simulink library "pacejka_trans"  (R2018b)
settings: Solver=ode45  StartTime=0.0  StopTime=10.0  RelTol=1e-3  EnableMultiTasking=on
undefined symbols (not defined in the file): DiscIntNeverNeededParam, par_TIR
libraries: simulink x2, $bdroot x1
(part 2 of 2)

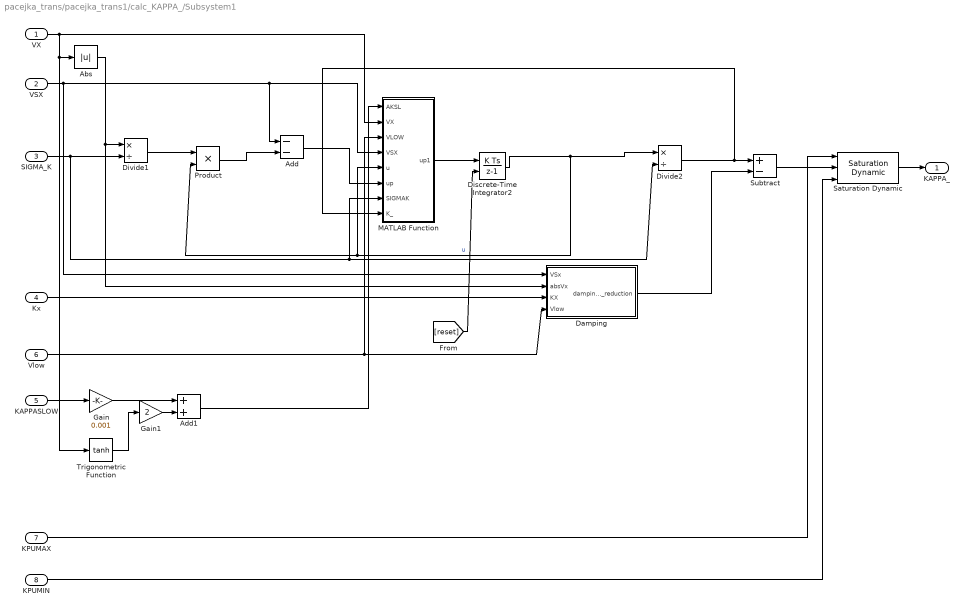
== system pacejka_trans/pacejka_trans1/calc_KAPPA_/Subsystem1 ==
  VX : Inport
  VSX : Inport  Port=2
  SIGMA_K : Inport  Port=3
  Kx : Inport  Port=4
  KAPPASLOW : Inport  Port=5
  Vlow : Inport  Port=6
  KPUMAX : Inport  Port=7
  KPUMIN : Inport  Port=8
  Abs : Abs
  Add : Sum  Inputs=--
  Add1 : Sum
  Damping : Subsystem
  Discrete-Time Integrator2 : DiscreteIntegrator  ExternalReset=sampled level  SampleTime=-1  ICPrevOutput=DiscIntNeverNeededParam  ICPrevScaledInput=DiscIntNeverNeededParam
  Divide1 : Product  Inputs=*/
  Divide2 : Product  Inputs=*/
  Gain : Gain  Gain=0.001
  Gain1 : Gain  Gain=2
  MATLAB Function : MATLAB Function  TreatAsAtomicUnit=on
  Product : Product  RndMeth=Zero
  Saturation Dynamic : simulink/Discontinuities/Saturation Dynamic  OutMin=[]  OutMax=[]  OutDataTypeStr=Inherit: Same as second input  OutDataType=fixdt(1, 16)  OutScaling=2^-10  DoSatur=off
  Subtract : Sum  Inputs=+-
  Trigonometric Function : Trigonometry  Operator=tanh
  KAPPA_ : Outport
  wires:
  Saturation Dynamic/1 -> KAPPA_/1
  KPUMIN/1 -> Saturation Dynamic/3
  KPUMAX/1 -> Saturation Dynamic/1
  MATLAB Function/1(up1) -> Discrete-Time Integrator2/1
  Add/1 -> MATLAB Function/6(up)
  Vlow/1 -> MATLAB Function/3(VLOW), Damping/4(Vlow)
  KAPPASLOW/1 -> Gain/1
  Kx/1 -> Damping/3(KX)
  Product/1 -> Add/2
  Divide1/1 -> Product/1
  Abs/1 -> Damping/2(absVx), Divide1/1
  VSX/1 -> MATLAB Function/4(VSX), Add/1, Damping/1(VSx)
  Discrete-Time Integrator2/1 -> Product/2, MATLAB Function/5(u), Divide2/1  "u"
  VX/1 -> Abs/1, Trigonometric Function/1, MATLAB Function/2(VX)
  SIGMA_K/1 -> Divide1/2, MATLAB Function/7(SIGMAK), Divide2/2
  Subtract/1 -> Saturation Dynamic/2
  Damping/1(damping_reduction) -> Subtract/2
  Divide2/1 -> Subtract/1, MATLAB Function/8(K_)
  Gain/1 -> Add1/1
  Trigonometric Function/1 -> Gain1/1
  Gain1/1 -> Add1/2
  Add1/1 -> MATLAB Function/1(AKSL)
  [reset] -> Discrete-Time Integrator2/2

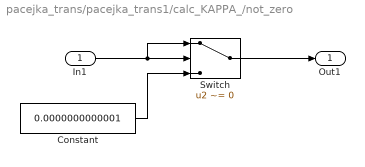
== system pacejka_trans/pacejka_trans1/calc_KAPPA_/not_zero ==
  In1 : Inport
  Constant : Constant  Value=0.0000000000001
  Switch : Switch  Criteria=u2 ~= 0
  Out1 : Outport
  wires:
  In1/1 -> Switch/1, Switch/2
  Constant/1 -> Switch/3
  Switch/1 -> Out1/1

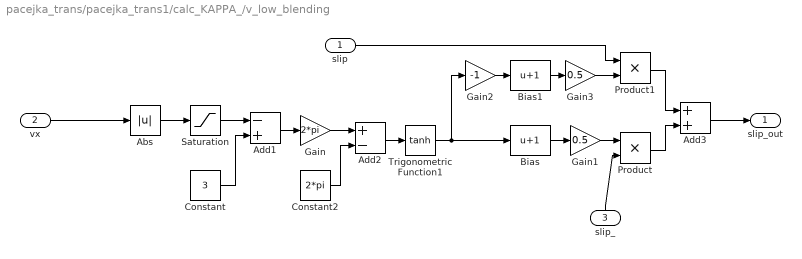
== system pacejka_trans/pacejka_trans1/calc_KAPPA_/v_low_blending  ==
  slip : Inport
  vx : Inport  Port=2
  slip_ : Inport  Port=3
  Abs : Abs
  Add1 : Sum  Inputs=-+
  Add2 : Sum  Inputs=+-
  Add3 : Sum
  Bias : Bias  Bias=1
  Bias1 : Bias  Bias=1
  Constant : Constant  Value=3
  Constant2 : Constant  Value=2*pi
  Gain : Gain  Gain=2*pi
  Gain1 : Gain  Gain=0.5
  Gain2 : Gain  Gain=-1
  Gain3 : Gain  Gain=0.5
  Product : Product
  Product1 : Product
  Saturation : Saturate  UpperLimit=3  LowerLimit=0
  Trigonometric Function1 : Trigonometry  Operator=tanh
  slip_out : Outport
  wires:
  Abs/1 -> Saturation/1
  Constant2/1 -> Add2/2
  Constant/1 -> Add1/2
  Gain/1 -> Add2/1
  Saturation/1 -> Add1/1
  Add2/1 -> Trigonometric Function1/1
  Add1/1 -> Gain/1
  Gain2/1 -> Bias1/1
  Gain1/1 -> Product/1
  Bias1/1 -> Gain3/1
  Product1/1 -> Add3/1
  Add3/1 -> slip_out/1
  Bias/1 -> Gain1/1
  Gain3/1 -> Product1/2
  Product/1 -> Add3/2
  slip/1 -> Product1/1
  Trigonometric Function1/1 -> Gain2/1, Bias/1
  slip_/1 -> Product/2
  vx/1 -> Abs/1

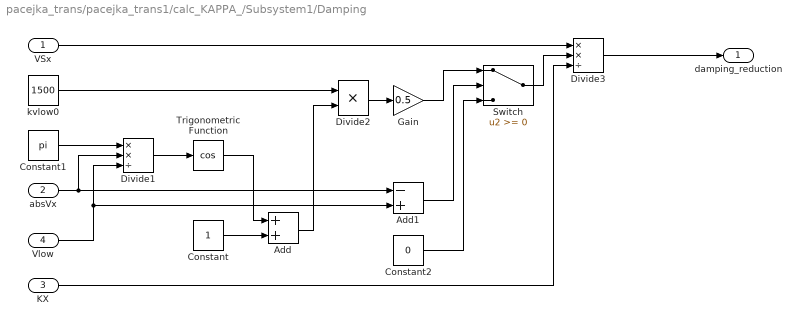
== system pacejka_trans/pacejka_trans1/calc_KAPPA_/Subsystem1/Damping ==
  VSx : Inport
  absVx : Inport  Port=2
  KX : Inport  Port=3
  Vlow : Inport  Port=4
  Add : Sum
  Add1 : Sum  Inputs=-+
  Constant : Constant
  Constant1 : Constant  Value=pi
  Constant2 : Constant  Value=0
  Divide1 : Product  Inputs=**/
  Divide2 : Product  Inputs=**
  Divide3 : Product  Inputs=**/
  Gain : Gain  Gain=0.5
  Switch : Switch
  Trigonometric Function : Trigonometry  Operator=cos
  kvlow0 : Constant  Value=1500
  damping_reduction : Outport
  wires:
  KX/1 -> Divide3/3
  Constant2/1 -> Switch/3
  Add1/1 -> Switch/2
  Divide3/1 -> damping_reduction/1
  Divide2/1 -> Gain/1
  VSx/1 -> Divide3/1
  Add/1 -> Divide2/2
  Divide1/1 -> Trigonometric Function/1
  Vlow/1 -> Add1/2, Divide1/3
  absVx/1 -> Add1/1, Divide1/2
  Constant1/1 -> Divide1/1
  Constant/1 -> Add/2
  Trigonometric Function/1 -> Add/1
  kvlow0/1 -> Divide2/1
  Gain/1 -> Switch/1
  Switch/1 -> Divide3/2

== matlab function pacejka_trans/pacejka_trans1/MATLAB Function ==
  data: RSTAT output; FZ input; OMEGA input; VX input; VSX output; VERTICAL_STIFFNESS input; FNOMIN input; UNLOADED_RADIUS input; BREFF input; DREFF input; FREFF input; RE output
function [RSTAT,VSX,RE] = longitudinal_slip_speed(FZ,OMEGA,VX,VERTICAL_STIFFNESS,FNOMIN,UNLOADED_RADIUS,BREFF,DREFF,FREFF)

RHO = FZ/VERTICAL_STIFFNESS;
RHOFZ0 = FNOMIN/VERTICAL_STIFFNESS;
RHOD = RHO/RHOFZ0;

RE = UNLOADED_RADIUS-RHOFZ0*(DREFF*atan(BREFF*RHOD)+FREFF*RHOD);
VSX = VX-OMEGA*RE;
RSTAT=UNLOADED_RADIUS-RHO;

end

== matlab function pacejka_trans/pacejka_trans1/calc_forces ==
  data: FZ input; KAPPA input; ALPHA input; GAMMA input; VX input; IP input; FNOMIN input; UNLOADED_RADIUS input; LONGVL input; LOADINDEX input; LFZO input; FX output; LCX input; LMUX input; LEX input; LKX input; LHX input; LVX input; LGAX input; LCY input; LMUY input; LEY input; LKY input; LHY input; LVY input; LGAY input; LTR input; LRES input; LGAZ input; LXAL input; LYKA input; LVYKA input; LS input; LMX input; LVMX input; LMY input; PCX1 input; PDX1 input; PDX2 input; PDX3 input; PEX1 input; PEX2 input; PEX3 input; PEX4 input; PKX1 input; PKX2 input; PKX3 input; PHX1 input; PHX2 input; PVX1 input; PVX2 input; RBX1 input; RBX2 input; RCX1 input; REX1 input; REX2 input; RHX1 input; QSX1 input; QSX2 input; QSX3 input; PCY1 input; PDY1 input; PDY2 input; PDY3 input; PEY1 input; PEY2 input; PEY3 input; PEY4 input; PKY1 input; PKY2 input; PKY3 input; PHY1 input; PHY2 input; PHY3 input; PVY1 input; PVY2 input; PVY3 input; PVY4 input; RBY1 input; RBY2 input; RBY3 input; RCY1 input; REY1 input; REY2 input; RHY1 input; RHY2 input; RVY1 input; RVY2 input; RVY3 input; RVY4 input; RVY5 input; RVY6 input; FY output; MX output; MY output; MZ output; QSY1 input; QSY2 input; QSY3 input; QSY4 input; QBZ1 input; QBZ2 input; QBZ3 input; QBZ4 input; QBZ5 input; QBZ9 input; QBZ10 input; QCZ1 input; QDZ1 input; QDZ2 input; QDZ3 input; QDZ4 input; QDZ6 input; QDZ7 input; QDZ8 input; QDZ9 input; QEZ1 input; QEZ2 input; QEZ3 input; QEZ4 input; QEZ5 input; QHZ1 input; QHZ2 input; QHZ3 input; QHZ4 input; SSZ1 input; SSZ2 input; SSZ3 input; SSZ4 input; T output; S output; Q output; c_kappa output; T_Z output; PIO input; PPX1 input; PPX2 input; PPX3 input; PPX4 input; PPY1 input; PPY2 input; PPY3 input; PPY4 input; QPZ1 input; KX output; DX output; DY output
function [FX,FY,MX,MY,MZ,T,S,Q,c_kappa,T_Z,KX,DX,DY] = magic_formula(...
    FZ, KAPPA, ALPHA, GAMMA, VX, IP,...                                         % INPUTS
    FNOMIN, UNLOADED_RADIUS, LONGVL, LOADINDEX,...                              % TIRE DATA
    LFZO,LCX,LMUX,LEX,LKX,LHX,LVX,LGAX,LCY,...                                  % SCALING FACTORS
    LMUY,LEY,LKY,LHY,LVY,LGAY,LTR,LRES,LGAZ,LXAL,LYKA,LVYKA,LS,...              % SCALING FACTORS
    LMX,LVMX,LMY,...                                                            % SCALING FACTORS
    PCX1,PDX1,PDX2,PDX3,PEX1,PEX2,PEX3,PEX4,PKX1,PKX2,PKX3,PHX1,...             % LONGITUDINAL COEFFICIENTS
    PHX2,PVX1,PVX2,RBX1,RBX2,RCX1,REX1,REX2,RHX1,...                            % LONGITUDINAL COEFFICIENTS
    QSX1,QSX2,QSX3,...                                                          % OVERTURNING COEFFICIENTS
    PCY1,PDY1,PDY2,PDY3,PEY1,PEY2,PEY3,PEY4,PKY1,...                            % LATERAL COEFFICIENTS
    PKY2,PKY3,PHY1,PHY2,PHY3,PVY1,PVY2,PVY3,PVY4,RBY1,RBY2,RBY3,RCY1,REY1,...   % LATERAL COEFFICIENTS
    REY2,RHY1,RHY2,RVY1,RVY2,RVY3,RVY4,RVY5,RVY6,...                            % LATERAL COEFFICIENTS
    QSY1,QSY2,QSY3,QSY4,...                                                     % ROLLING COEFFICIENTS
    QBZ1, QBZ2, QBZ3, QBZ4, QBZ5, QBZ9, QBZ10, QCZ1, QDZ1,...                   % ALIGNING COEFFICIENTS
    QDZ2,QDZ3,QDZ4,QDZ6,QDZ7,QDZ8,QDZ9,QEZ1,QEZ2,QEZ3,QEZ4,QEZ5,...             % ALIGNING COEFFICIENTS
    QHZ1,QHZ2,QHZ3,QHZ4,SSZ1,SSZ2,SSZ3,SSZ4,...                                 % ALIGNING COEFFICIENTS
    PIO, PPX1, PPX2, PPX3, PPX4, PPY1, PPY2, PPY3, PPY4, QPZ1)                  % PRESSURE COEFFICIENTS

%% INITIALISIERUNG

% Referenzgeschwindigkeit auf diejenige aus dem Reifenfile festlegen
VREF = LONGVL;

% calculate normalized vertical load increment dFZ
FNOMIN_ = FNOMIN.*LFZO;
dFZ = (FZ-FNOMIN_)./FNOMIN_;

% calculate normalized change in inflation pressure dPI
dPI = (IP-PIO)./PIO;

%% LONGITUDINAL

% pure slip
GAMMAX = GAMMA.*LGAX;
SHX = (PHX1+PHX2.*dFZ).*LHX;
SVX = FZ.*(PVX1+PVX2.*dFZ).*LVX.*LMUX;
KAPPAX = KAPPA+SHX;
MUX = (PDX1+PDX2.*dFZ).*(1-PDX3.*GAMMAX.^2).*LMUX.*(1+PPX3.*dPI+PPX4.*dPI.^2);
CX = PCX1.*LCX;
DX = MUX.*FZ;
EX = (PEX1+PEX2.*dFZ+PEX3.*dFZ.^2).*(1-PEX4.*sign(KAPPAX)).*LEX;
EX(EX>1) = 1;
KX = FZ.*(PKX1+PKX2.*dFZ).*exp(PKX3.*dFZ).*LKX.*(1+PPX1.*dPI+PPX2.*dPI.^2);
BX = KX./(CX.*DX);
FX0 = DX.*sin(CX.*atan(BX.*KAPPAX-EX.*(BX.*KAPPAX-atan(BX.*KAPPAX))))+SVX;

% combined slip
SHXA = RHX1;
ALPHAS = ALPHA+SHXA;
BXA = RBX1.*cos(atan(RBX2.*KAPPA)).*LXAL;
CXA = RCX1;
EXA = REX1+REX2.*dFZ;
GXA0 = cos(CXA.*atan(BXA.*SHXA-EXA.*(BXA.*SHXA-atan(BXA.*SHXA))));
GXA = cos(CXA.*atan(BXA.*ALPHAS-EXA.*(BXA.*ALPHAS-atan(BXA.*ALPHAS))))./GXA0;
FX = GXA.*FX0;

%% LATERAL

% pure slip
GAMMAY = GAMMA.*LGAY;
SHY = (PHY1+PHY2.*dFZ).*LHY+PHY3.*GAMMAY;
ALPHAY = ALPHA+SHY;
MUY = (PDY1+PDY2.*dFZ).*(1-PDY3.*GAMMAY.^2).*LMUY.*(1+PPY3.*dPI+PPY4.*dPI.^2);
SVY = FZ.*((PVY1+PVY2.*dFZ).*LVY+(PVY3+PVY4.*dFZ).*GAMMAY).*LMUY;
DY = MUY.*FZ;
CY = PCY1.*LCY;
EY = (PEY1+PEY2.*dFZ).*(1-(PEY3+PEY4.*GAMMAY).*sign(ALPHAY)).*LEY;
EY(EY>1) = 1;
KY = PKY1.*FNOMIN.*sin(2.*atan(FZ./(PKY2.*FNOMIN.*LFZO.*(1+PPY2.*dPI)))).*(1-PKY3.*abs(GAMMAY)).*LFZO.*LKY.*(1+PPY1.*dPI);
BY = KY./(CY.*DY);
FY0 = DY.*sin(CY.*atan(BY.*ALPHAY-EY.*(BY.*ALPHAY-atan(BY.*ALPHAY))))+SVY;

%combined slip
SHYK = RHY1+RHY2.*dFZ;
KAPPAS = KAPPA+SHYK;
BYK = RBY1.*cos(atan(RBY2.*(ALPHA-RBY3))).*LYKA;
CYK = RCY1;
EYK = REY1+REY2.*dFZ;
DVYK = MUY.*FZ.*(RVY1+RVY2.*dFZ+RVY3.*GAMMA).*cos(atan(RVY4.*ALPHA));
SVYK = DVYK.*sin(RVY5.*atan(RVY6.*KAPPA)).*LVYKA;
GYK0 = cos(CYK.*atan(BYK.*SHYK-EYK.*(BYK.*SHYK-atan(BYK.*SHYK))));
GYK = cos(CYK.*atan(BYK.*KAPPAS-EYK.*(BYK.*KAPPAS-atan(BYK.*KAPPAS))))./GYK0;
FY = GYK.*FY0+SVYK;

%% ALIGNING TORQUE

% pure Slip
GAMMAZ = GAMMA.*LGAZ;
SHT = QHZ1+QHZ2.*dFZ+(QHZ3+QHZ4.*dFZ).*GAMMAZ;
ALPHAT = ALPHA+SHT;
BT = (QBZ1+QBZ2.*dFZ+QBZ3.*dFZ.^2).*(1+QBZ4.*GAMMAZ+QBZ5.*abs(GAMMAZ)).*LKY./LMUY;
CT = QCZ1;
DT = FZ.*(QDZ1+QDZ2.*dFZ).*(1+QDZ3.*GAMMAZ+QDZ4.*GAMMAZ.^2).*(UNLOADED_RADIUS./FNOMIN).*LTR.*(1-QPZ1.*dPI);
ET = (QEZ1+QEZ2.*dFZ+QEZ3.*dFZ.^2).*(1+(QEZ4+QEZ5.*GAMMAZ).*2./pi.*atan(BT.*CT.*ALPHAT));
ET(ET>1) = 1;
% T = DT.*cos(CT.*atan(BT.*ALPHAT-ET.*(BT.*ALPHAT-atan(BT.*ALPHAT)))).*cos(ALPHA); % pneumatic trail
SHR = SHY+SVY./KY;
ALPHAR = ALPHA+SHR;
DR = FZ.*((QDZ6+QDZ7.*dFZ).*LRES+(QDZ8+QDZ9.*dFZ).*GAMMAZ).*UNLOADED_RADIUS.*LMUY;
BR = QBZ9.*LKY./LMUY+QBZ10.*BY.*CY;
% MZR = DR.*cos(atan(BR.*ALPHAR)).*cos(ALPHA);
% MZ0 = -T.*FY0+MZR;
% KZ = -T.*KY; % approximation for the aligning moment stiffness

%%% Combined Slip
ALPHATEQ = atan(sqrt((tan(ALPHAT)).^2+(KX./KY).^2.*KAPPA.^2)).*sign(ALPHAT);
ALPHAREQ = atan(sqrt((tan(ALPHAR)).^2+(KX./KY).^2.*KAPPA.^2)).*sign(ALPHAR);
T = DT.*cos(CT.*atan(BT.*ALPHATEQ-ET.*(BT.*ALPHATEQ-atan(BT.*ALPHATEQ)))).*cos(ALPHA);
FY_ = FY-SVYK;
MZR = DR.*cos(atan(BR.*ALPHAREQ)).*cos(ALPHA);
S = (SSZ1+SSZ2.*(FY./FNOMIN)+(SSZ3+SSZ4.*dFZ).*GAMMA).*UNLOADED_RADIUS.*LS;
MZ = -T.*FY_+MZR+S.*FX;

%% OVERTURNING MOMENT
Q = UNLOADED_RADIUS.*(QSX1.*LVMX+(-QSX2.*GAMMA+QSX3.*FY./FNOMIN).*LMX);
MX = Q.*FZ;

%% ROLLING RESISTANCE TORQUE

% create tire load capacity depending on tire load index
load_capacity = [62 : 120; 265, 272, 280, 290, 300, 307, 315, 325, 335, 345, 355, 365, 375, ...
    387, 400, 412, 425, 437, 450, 462, 475, 487, 500, 515, 530, 545, 560, 580, 600, 615, 630, ...
    650, 670, 690, 710, 730, 750, 775, 800, 825, 850, 875, 900, 925, 950, 975, 1000, 1030, 1060, ...
    1090, 1120, 1150, 1180, 1215, 1250, 1285, 1320, 1360, 1400]; % [load index; capacity in [kg]]

% unit conversion: [kg] -> [N]
load_capacity(2, :) = load_capacity(2, :) * 9.81;

% get reference value of load_capacity (80% of maximum load capacity)
[~, index] = min(abs(load_capacity(1, :) - LOADINDEX));
FZ_ref = load_capacity(2, index) * 0.8;

% set reference inflation pressure (210 kPa for the tire labeling)
IP_ref = 210;

% use Michelin formula to calculate the rolling resistance scaling factor depending on inflation pressure and with better approximation of wheel load
IP_ALPHA = -0.4;
IP_BETA = 0.85;

if QSY1==0 && QSY2==0
    MY = UNLOADED_RADIUS.*(SVX+KX.*SHX).*sign(VX);
else
%     MY = -UNLOADED_RADIUS.*FZ.*(QSY1+QSY2.*FX./FNOMIN+QSY3.*abs(VX./VREF)+QSY4.*(VX./VREF).^4).*sign(VX).*LMY; % original formula
    MY = -UNLOADED_RADIUS.*FZ_ref.*(QSY1+QSY2.*FX./FNOMIN+QSY3.*abs(VX./VREF)+QSY4.*(VX./VREF).^4).*sign(VX).*LMY.*(IP./IP_ref).^IP_ALPHA.*(FZ./FZ_ref).^IP_BETA; % modified Michelin formula
end

MY(abs(VX)<0.008) = 0;

%% ERWEITERUNGEN LENKMODELL

% Hebelarme
if QSY1==0 && QSY2==0
    T_Z = 0;
else
    T_Z = -UNLOADED_RADIUS.*(QSY1+QSY2.*FX./FNOMIN+QSY3.*abs(VX./VREF)+QSY4.*(VX./VREF).^4).*sign(VX).*LMY;
end

% Brechnung der Laengskraftabhaengigkeit vom Schlupf
KAPPA__ = KAPPA+0.001;

% pure slip
% GAMMAX = GAMMA.*LGAX;
% SHX = (PHX1+PHX2.*dFZ).*LHX;
% SVX = FZ.*(PVX1+PVX2.*dFZ).*LVX.*LMUX;
KAPPAX__ = KAPPA__+SHX;
% MUX = (PDX1+PDX2.*dFZ).*(1-PDX3.*GAMMAX.^2).*LMUX.*(1+PPX3.*dPI+PPX4.*dPI.^2);
% CX = PCX1.*LCX;
% DX = MUX.*FZ;
EX__ = (PEX1+PEX2.*dFZ+PEX3.*dFZ.^2).*(1-PEX4.*sign(KAPPAX__)).*LEX;
EX__(EX__>1) = 1;
% KX = FZ.*(PKX1+PKX2.*dFZ).*exp(PKX3.*dFZ).*LKX.*(1+PPX1.*dPI+PPX2.*dPI.^2);
% BX = KX./(CX.*DX);
FX0__ = DX.*sin(CX.*atan(BX.*KAPPAX__-EX__.*(BX.*KAPPAX__-atan(BX.*KAPPAX__))))+SVX;

% combined slip
% SHXA = RHX1;
% ALPHAS = ALPHA+SHXA;
BXA__ = RBX1.*cos(atan(RBX2.*KAPPA__)).*LXAL;
% CXA = RCX1;
% EXA = REX1+REX2.*dFZ;
GXA0__ = cos(CXA.*atan(BXA__.*SHXA-EXA.*(BXA__.*SHXA-atan(BXA__.*SHXA))));
GXA__ = cos(CXA.*atan(BXA__.*ALPHAS-EXA.*(BXA__.*ALPHAS-atan(BXA__.*ALPHAS))))./GXA0__;
FX__ = GXA__.*FX0__;

c_kappa = (FX__-FX)./0.001;

end

== matlab function pacejka_trans/pacejka_trans1/calc_trans_fac ==
  data: GAMMA input; FZ input; IP input; FNOMIN input; UNLOADED_RADIUS input; FZMIN input; LFZO input; LSGAL input; LSGKP input; LKX input; LKY input; LGAX input; LGAY input; LMUX input; LMUY input; PTX1 input; PTX2 input; PTX3 input; PTY1 input; PTY2 input; PKY1 input; PKY2 input; PKY3 input; PKX1 input; PKX2 input; PKX3 input; PDX1 input; PDX2 input; PDX3 input; PDY1 input; PDY2 input; PDY3 input; SIGMA_A output; SIGMA_K output; KX output; KAPPASLOW output; ALPHASLOW output; PIO input; PPX1 input; PPX2 input; PPX3 input; PPX4 input; PPY1 input; PPY2 input; PPY3 input; PPY4 input
function [SIGMA_A,SIGMA_K,KX,KAPPASLOW,ALPHASLOW] = stretched_string(...
    GAMMA, FZ, IP, ...
    FNOMIN, UNLOADED_RADIUS, FZMIN, ...
    LFZO, LSGAL, LSGKP, LKX, LKY, LGAX, LGAY, LMUX, LMUY, ...
    PTX1, PTX2, PTX3,  PTY1, PTY2, PKY1, PKY2, PKY3, PKX1, PKX2, PKX3, PDX1, PDX2, PDX3, PDY1, PDY2, PDY3, ...
    PIO, PPX1, PPX2, PPX3, PPX4, PPY1, PPY2, PPY3, PPY4)

%% INITIALIZATION

% calculate normalized vertical load increment dFZ
FNOMIN_ = FNOMIN.*LFZO;
dFZ = (FZ-FNOMIN_)./FNOMIN_;

% calculate normalized change in inflation pressure dPI
dPI = (IP-PIO)./PIO;

%% TRANSIENT BEHAVIOR

SIGMA_K = FZ*(PTX1+PTX2*dFZ)*exp(-PTX3*dFZ)*(UNLOADED_RADIUS/FNOMIN)*LSGKP;
SIGMA_A = PTY1*sin(2*atan(FZ/(PTY2*FNOMIN*LFZO)))*(1-PKY3*abs(GAMMA))*UNLOADED_RADIUS*LFZO*LSGAL;

%% LIMIT RELAXATION LENGTHS FOR VALID BEHAVIOUR

if FZ<FZMIN
    dFZ = (FZMIN-FNOMIN_)/FNOMIN_;
    SIGMA_K = FZMIN*(PTX1+PTX2*dFZ)*exp(-PTX3*dFZ)*(UNLOADED_RADIUS/FNOMIN)*LSGKP;
    SIGMA_A = PTY1*sin(2*atan(FZMIN/(PTY2*FNOMIN*LFZO)))*(1-PKY3*abs(GAMMA))*UNLOADED_RADIUS*LFZO*LSGAL;
end

%% LIMIT RELAXATION LENGTHS FOR NUMERICAL STABILITY

SIGMA_K(SIGMA_K < 0.0176) = 0.0176;
SIGMA_A(SIGMA_A < 0.02) = 0.02;

GAMMAX = GAMMA.*LGAX;
KX = FZ.*(PKX1+PKX2.*dFZ).*exp(PKX3.*dFZ).*LKX.*(1+PPX1.*dPI+PPX2.*dPI.^2);
MUX = (PDX1+PDX2.*dFZ).*(1-PDX3.*GAMMAX.^2).*LMUX.*(1+PPX3.*dPI+PPX4.*dPI.^2);
DX = MUX.*FZ;
KAPPASLOW = 3.*DX./KX;

GAMMAY = GAMMA.*LGAY;
KY = PKY1.*FNOMIN.*sin(2.*atan(FZ./(PKY2.*FNOMIN.*LFZO.*(1+PPY2.*dPI)))).*(1-PKY3.*abs(GAMMAY)).*LFZO.*LKY.*(1+PPY1.*dPI);
MUY = (PDY1+PDY2.*dFZ).*(1-PDY3.*GAMMAY.^2).*LMUY.*(1+PPY3.*dPI+PPY4.*dPI.^2);
DY=MUY.*FZ;
ALPHASLOW = 3.*DY./KY;

end

== matlab function pacejka_trans/pacejka_trans1/calc_ALPHA/Subsystem1/MATLAB Function ==
  data: ALPHASL input; VX input; VLOW input; VSY input; v input; vp input; vp1 output; SIGMAA input; ALPHAreq_ input
function vp1 = fcn(ALPHASL,VX,VLOW,VSY,v,vp,SIGMAA, ALPHAreq_)
%#codegen

if abs(ALPHAreq_)>ALPHASL && abs(VX)<VLOW && (VSY+abs(VX)*v/SIGMAA)*v<0
    vp1=0;
else
    vp1=vp;
end

== matlab function pacejka_trans/pacejka_trans1/calc_KAPPA_/Subsystem1/MATLAB Function ==
  data: AKSL input; VX input; VLOW input; VSX input; u input; up input; up1 output; SIGMAK input; K_ input
function up1 = fcn(AKSL,VX,VLOW,VSX,u,up,SIGMAK, K_)
%#codegen

if abs(K_)>AKSL && abs(VX)<VLOW && (VSX+abs(VX)*u/SIGMAK)*u<0
    up1=0;
else
    up1=up;
end
